simulink model "Lombardy"  (Simulink 7.9)
settings: Solver=ode45  StartTime=0.0  StopTime=10.0  RelTol=1e-3
undefined symbols (not defined in the file or in its folder): f_NODE01, f_NODE02, f_NODE03, f_NODE04, f_NODE05, f_NODE06, f_NODE07, f_NODE08, f_NODE09, f_NODE10, f_NODE11, f_NODE12, f_NODE13, f_NODE14, f_NODE15, f_NODE16, f_NODE17, f_NODE18, f_NODE19, f_NODE20, f_NODE21, f_NODE22, f_NODE23, f_NODE24, f_NODE25, f_NODE26, f_NODE27, f_NODE28, f_NODE29, f_NODE30, f_NODE31, f_NODE32, r_NODE01, r_NODE02, r_NODE03, r_NODE04, r_NODE05, r_NODE06, r_NODE07, r_NODE08, r_NODE09, r_NODE10, r_NODE11, r_NODE12, r_NODE13, r_NODE14, r_NODE15, r_NODE16, r_NODE17, r_NODE18, r_NODE19, r_NODE20, r_NODE21, r_NODE22, r_NODE23, r_NODE24, r_NODE25, r_NODE26, r_NODE27, r_NODE28 ... (+36)
(part 1 of 2)
settings Model: Creator=lanalfa  LastModifiedBy=lanalfa

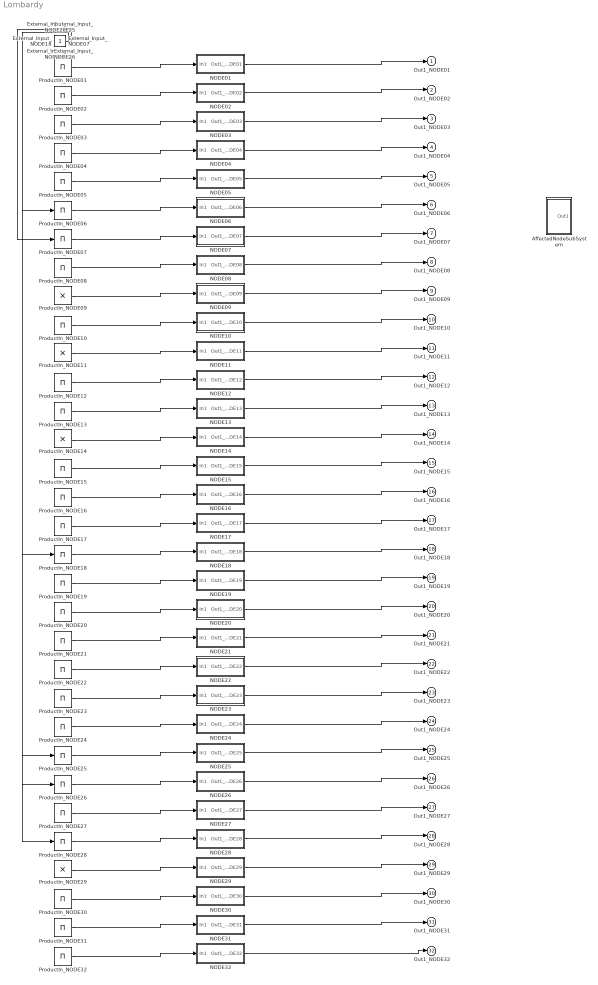
== system Lombardy ==
  AffectedNodeSubSystem : Subsystem
  External_Input_NODE06 : Constant
  External_Input_NODE07 : Constant
  External_Input_NODE{18,25..26,28} (4 alike) : Constant
  NODE01 : Subsystem
  NODE02 : Subsystem
  NODE03 : Subsystem
  NODE04 : Subsystem
  NODE05 : Subsystem
  NODE06 : Subsystem
  NODE07 : Subsystem
  NODE08 : Subsystem
  NODE09 : Subsystem
  NODE10 : Subsystem
  NODE11 : Subsystem
  NODE12 : Subsystem
  NODE13 : Subsystem
  NODE14 : Subsystem
  NODE15 : Subsystem
  NODE16 : Subsystem
  NODE17 : Subsystem
  NODE18 : Subsystem
  NODE19 : Subsystem
  NODE20 : Subsystem
  NODE21 : Subsystem
  NODE22 : Subsystem
  NODE23 : Subsystem
  NODE24 : Subsystem
  NODE25 : Subsystem
  NODE26 : Subsystem
  NODE27 : Subsystem
  NODE28 : Subsystem
  NODE29 : Subsystem
  NODE30 : Subsystem
  NODE31 : Subsystem
  NODE32 : Subsystem
  ProductIn_NODE01 : Product  Inputs=1  SaturateOnIntegerOverflow=on  RndMeth=Zero  InputSameDT=on
  ProductIn_NODE02 : Product  Inputs=1  SaturateOnIntegerOverflow=on  RndMeth=Zero  InputSameDT=on
  ProductIn_NODE03 : Product  Inputs=1  SaturateOnIntegerOverflow=on  RndMeth=Zero  InputSameDT=on
  ProductIn_NODE04 : Product  Inputs=1  SaturateOnIntegerOverflow=on  RndMeth=Zero  InputSameDT=on
  ProductIn_NODE05 : Product  Inputs=1  SaturateOnIntegerOverflow=on  RndMeth=Zero  InputSameDT=on
  ProductIn_NODE06 : Product  Inputs=1  SaturateOnIntegerOverflow=on  RndMeth=Zero  InputSameDT=on
  ProductIn_NODE07 : Product  Inputs=1  SaturateOnIntegerOverflow=on  RndMeth=Zero  InputSameDT=on
  ProductIn_NODE08 : Product  Inputs=1  SaturateOnIntegerOverflow=on  RndMeth=Zero  InputSameDT=on
  ProductIn_NODE09 : Product  SaturateOnIntegerOverflow=on  RndMeth=Zero  InputSameDT=on
  ProductIn_NODE{10,12..13,15..28,30..32} (20 alike) : Product  Inputs=1  SaturateOnIntegerOverflow=on  RndMeth=Zero  InputSameDT=on
  ProductIn_NODE11 : Product  SaturateOnIntegerOverflow=on  RndMeth=Zero  InputSameDT=on
  ProductIn_NODE14 : Product  Inputs=4  SaturateOnIntegerOverflow=on  RndMeth=Zero  InputSameDT=on
  ProductIn_NODE29 : Product  SaturateOnIntegerOverflow=on  RndMeth=Zero  InputSameDT=on
  Out1_NODE01 : Outport
  Out1_NODE02 : Outport  Port=2
  Out1_NODE03 : Outport  Port=3
  Out1_NODE04 : Outport  Port=4
  Out1_NODE05 : Outport  Port=5
  Out1_NODE06 : Outport  Port=6
  Out1_NODE07 : Outport  Port=7
  Out1_NODE08 : Outport  Port=8
  Out1_NODE09 : Outport  Port=9
  Out1_NODE10 : Outport  Port=10
  Out1_NODE11 : Outport  Port=11
  Out1_NODE12 : Outport  Port=12
  Out1_NODE13 : Outport  Port=13
  Out1_NODE14 : Outport  Port=14
  Out1_NODE15 : Outport  Port=15
  Out1_NODE16 : Outport  Port=16
  Out1_NODE17 : Outport  Port=17
  Out1_NODE18 : Outport  Port=18
  Out1_NODE19 : Outport  Port=19
  Out1_NODE20 : Outport  Port=20
  Out1_NODE21 : Outport  Port=21
  Out1_NODE22 : Outport  Port=22
  Out1_NODE23 : Outport  Port=23
  Out1_NODE24 : Outport  Port=24
  Out1_NODE25 : Outport  Port=25
  Out1_NODE26 : Outport  Port=26
  Out1_NODE27 : Outport  Port=27
  Out1_NODE28 : Outport  Port=28
  Out1_NODE29 : Outport  Port=29
  Out1_NODE30 : Outport  Port=30
  Out1_NODE31 : Outport  Port=31
  Out1_NODE32 : Outport  Port=32
  wires:
  ProductIn_NODE01/1 -> NODE01/1(In1)
  NODE01/1(Out1_NODE01) -> Out1_NODE01/1
  ProductIn_NODE02/1 -> NODE02/1(In1)
  NODE02/1(Out1_NODE02) -> Out1_NODE02/1
  ProductIn_NODE03/1 -> NODE03/1(In1)
  NODE03/1(Out1_NODE03) -> Out1_NODE03/1
  ProductIn_NODE04/1 -> NODE04/1(In1)
  NODE04/1(Out1_NODE04) -> Out1_NODE04/1
  ProductIn_NODE05/1 -> NODE05/1(In1)
  NODE05/1(Out1_NODE05) -> Out1_NODE05/1
  ProductIn_NODE06/1 -> NODE06/1(In1)
  NODE06/1(Out1_NODE06) -> Out1_NODE06/1
  ProductIn_NODE07/1 -> NODE07/1(In1)
  NODE07/1(Out1_NODE07) -> Out1_NODE07/1
  ProductIn_NODE08/1 -> NODE08/1(In1)
  NODE08/1(Out1_NODE08) -> Out1_NODE08/1
  ProductIn_NODE09/1 -> NODE09/1(In1)
  NODE09/1(Out1_NODE09) -> Out1_NODE09/1
  ProductIn_NODE10/1 -> NODE10/1(In1)
  NODE10/1(Out1_NODE10) -> Out1_NODE10/1
  ProductIn_NODE11/1 -> NODE11/1(In1)
  NODE11/1(Out1_NODE11) -> Out1_NODE11/1
  ProductIn_NODE12/1 -> NODE12/1(In1)
  NODE12/1(Out1_NODE12) -> Out1_NODE12/1
  ProductIn_NODE13/1 -> NODE13/1(In1)
  NODE13/1(Out1_NODE13) -> Out1_NODE13/1
  ProductIn_NODE14/1 -> NODE14/1(In1)
  NODE14/1(Out1_NODE14) -> Out1_NODE14/1
  ProductIn_NODE15/1 -> NODE15/1(In1)
  NODE15/1(Out1_NODE15) -> Out1_NODE15/1
  ProductIn_NODE16/1 -> NODE16/1(In1)
  NODE16/1(Out1_NODE16) -> Out1_NODE16/1
  ProductIn_NODE17/1 -> NODE17/1(In1)
  NODE17/1(Out1_NODE17) -> Out1_NODE17/1
  ProductIn_NODE18/1 -> NODE18/1(In1)
  NODE18/1(Out1_NODE18) -> Out1_NODE18/1
  ProductIn_NODE19/1 -> NODE19/1(In1)
  NODE19/1(Out1_NODE19) -> Out1_NODE19/1
  ProductIn_NODE20/1 -> NODE20/1(In1)
  NODE20/1(Out1_NODE20) -> Out1_NODE20/1
  ProductIn_NODE21/1 -> NODE21/1(In1)
  NODE21/1(Out1_NODE21) -> Out1_NODE21/1
  ProductIn_NODE22/1 -> NODE22/1(In1)
  NODE22/1(Out1_NODE22) -> Out1_NODE22/1
  ProductIn_NODE23/1 -> NODE23/1(In1)
  NODE23/1(Out1_NODE23) -> Out1_NODE23/1
  ProductIn_NODE24/1 -> NODE24/1(In1)
  NODE24/1(Out1_NODE24) -> Out1_NODE24/1
  ProductIn_NODE25/1 -> NODE25/1(In1)
  NODE25/1(Out1_NODE25) -> Out1_NODE25/1
  ProductIn_NODE26/1 -> NODE26/1(In1)
  NODE26/1(Out1_NODE26) -> Out1_NODE26/1
  ProductIn_NODE27/1 -> NODE27/1(In1)
  NODE27/1(Out1_NODE27) -> Out1_NODE27/1
  ProductIn_NODE28/1 -> NODE28/1(In1)
  NODE28/1(Out1_NODE28) -> Out1_NODE28/1
  ProductIn_NODE29/1 -> NODE29/1(In1)
  NODE29/1(Out1_NODE29) -> Out1_NODE29/1
  ProductIn_NODE30/1 -> NODE30/1(In1)
  NODE30/1(Out1_NODE30) -> Out1_NODE30/1
  ProductIn_NODE31/1 -> NODE31/1(In1)
  NODE31/1(Out1_NODE31) -> Out1_NODE31/1
  ProductIn_NODE32/1 -> NODE32/1(In1)
  NODE32/1(Out1_NODE32) -> Out1_NODE32/1
  External_Input_NODE06/1 -> ProductIn_NODE06/1
  External_Input_NODE07/1 -> ProductIn_NODE07/1
  External_Input_NODE18/1 -> ProductIn_NODE18/1
  External_Input_NODE25/1 -> ProductIn_NODE25/1
  External_Input_NODE26/1 -> ProductIn_NODE26/1
  External_Input_NODE28/1 -> ProductIn_NODE28/1

== system Lombardy/AffectedNodeSubSystem ==
  Pulse Generator_NODE : DiscretePulseGenerator  PulseType=Time based  Period=1  PulseWidth=60  PhaseDelay=0.4
  Out1 : Outport
  wires:
  Pulse Generator_NODE/1 -> Out1/1

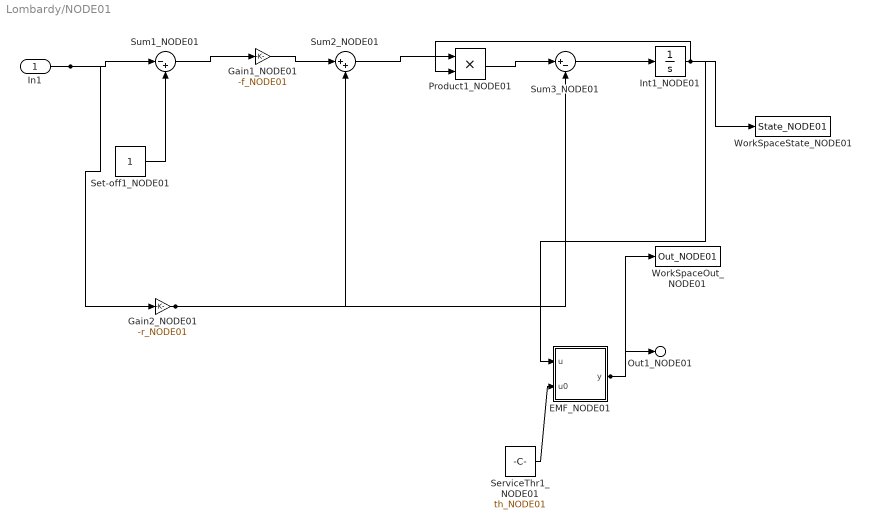
== system Lombardy/NODE01 ==
  In1 : Inport
  EMF_NODE01 : MATLAB Function  TreatAsAtomicUnit=on
  Gain1_NODE01 : Gain  Gain=-f_NODE01  SaturateOnIntegerOverflow=on  OutDataTypeStr=Inherit: Same as input  ParamDataTypeStr=Inherit: Same as input
  Gain2_NODE01 : Gain  Gain=-r_NODE01  SaturateOnIntegerOverflow=on  OutDataTypeStr=Inherit: Same as input  ParamDataTypeStr=Inherit: Same as input
  Int1_NODE01 : Integrator  InitialCondition=1
  Product1_NODE01 : Product  SaturateOnIntegerOverflow=on  RndMeth=Zero  InputSameDT=on
  ServiceThr1_NODE01 : Constant  Value=th_NODE01
  Set-off1_NODE01 : Constant
  Sum1_NODE01 : Sum  Inputs=|-+  SaturateOnIntegerOverflow=on  InputSameDT=on
  Sum2_NODE01 : Sum  Inputs=|++  SaturateOnIntegerOverflow=on  InputSameDT=on
  Sum3_NODE01 : Sum  Inputs=|+-  SaturateOnIntegerOverflow=on  InputSameDT=on
  WorkSpaceOut_NODE01 : ToWorkspace  VariableName=Out_NODE01
  WorkSpaceState_NODE01 : ToWorkspace  VariableName=State_NODE01
  Out1_NODE01 : Outport
  wires:
  In1/1 -> Gain2_NODE01/1, Sum1_NODE01/1
  Set-off1_NODE01/1 -> Sum1_NODE01/2
  Sum1_NODE01/1 -> Gain1_NODE01/1
  Gain1_NODE01/1 -> Sum2_NODE01/1
  Gain2_NODE01/1 -> Sum2_NODE01/2, Sum3_NODE01/2
  Sum2_NODE01/1 -> Product1_NODE01/1
  Product1_NODE01/1 -> Sum3_NODE01/1
  Int1_NODE01/1 -> Product1_NODE01/2, EMF_NODE01/1(u), WorkSpaceState_NODE01/1
  Sum3_NODE01/1 -> Int1_NODE01/1
  ServiceThr1_NODE01/1 -> EMF_NODE01/2(u0)
  EMF_NODE01/1(y) -> Out1_NODE01/1, WorkSpaceOut_NODE01/1

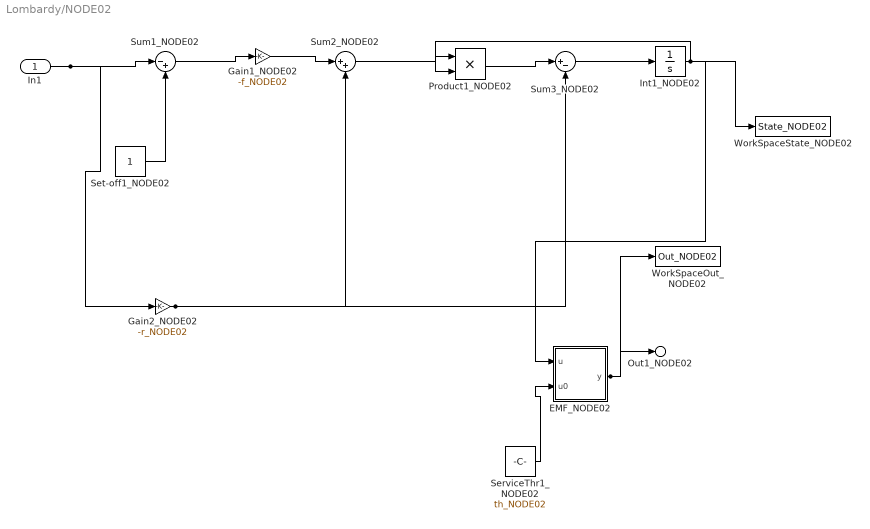
== system Lombardy/NODE02 ==
  In1 : Inport
  EMF_NODE02 : MATLAB Function  TreatAsAtomicUnit=on
  Gain1_NODE02 : Gain  Gain=-f_NODE02  SaturateOnIntegerOverflow=on  OutDataTypeStr=Inherit: Same as input  ParamDataTypeStr=Inherit: Same as input
  Gain2_NODE02 : Gain  Gain=-r_NODE02  SaturateOnIntegerOverflow=on  OutDataTypeStr=Inherit: Same as input  ParamDataTypeStr=Inherit: Same as input
  Int1_NODE02 : Integrator  InitialCondition=1
  Product1_NODE02 : Product  SaturateOnIntegerOverflow=on  RndMeth=Zero  InputSameDT=on
  ServiceThr1_NODE02 : Constant  Value=th_NODE02
  Set-off1_NODE02 : Constant
  Sum1_NODE02 : Sum  Inputs=|-+  SaturateOnIntegerOverflow=on  InputSameDT=on
  Sum2_NODE02 : Sum  Inputs=|++  SaturateOnIntegerOverflow=on  InputSameDT=on
  Sum3_NODE02 : Sum  Inputs=|+-  SaturateOnIntegerOverflow=on  InputSameDT=on
  WorkSpaceOut_NODE02 : ToWorkspace  VariableName=Out_NODE02
  WorkSpaceState_NODE02 : ToWorkspace  VariableName=State_NODE02
  Out1_NODE02 : Outport
  wires:
  In1/1 -> Gain2_NODE02/1, Sum1_NODE02/1
  Set-off1_NODE02/1 -> Sum1_NODE02/2
  Sum1_NODE02/1 -> Gain1_NODE02/1
  Gain1_NODE02/1 -> Sum2_NODE02/1
  Gain2_NODE02/1 -> Sum2_NODE02/2, Sum3_NODE02/2
  Sum2_NODE02/1 -> Product1_NODE02/1
  Product1_NODE02/1 -> Sum3_NODE02/1
  Int1_NODE02/1 -> Product1_NODE02/2, EMF_NODE02/1(u), WorkSpaceState_NODE02/1
  Sum3_NODE02/1 -> Int1_NODE02/1
  ServiceThr1_NODE02/1 -> EMF_NODE02/2(u0)
  EMF_NODE02/1(y) -> Out1_NODE02/1, WorkSpaceOut_NODE02/1

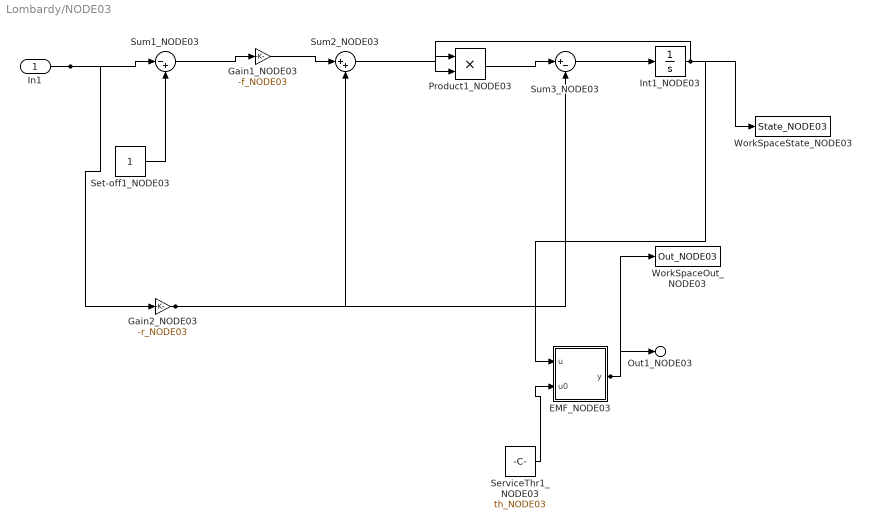
== system Lombardy/NODE03 ==
  In1 : Inport
  EMF_NODE03 : MATLAB Function  TreatAsAtomicUnit=on
  Gain1_NODE03 : Gain  Gain=-f_NODE03  SaturateOnIntegerOverflow=on  OutDataTypeStr=Inherit: Same as input  ParamDataTypeStr=Inherit: Same as input
  Gain2_NODE03 : Gain  Gain=-r_NODE03  SaturateOnIntegerOverflow=on  OutDataTypeStr=Inherit: Same as input  ParamDataTypeStr=Inherit: Same as input
  Int1_NODE03 : Integrator  InitialCondition=1
  Product1_NODE03 : Product  SaturateOnIntegerOverflow=on  RndMeth=Zero  InputSameDT=on
  ServiceThr1_NODE03 : Constant  Value=th_NODE03
  Set-off1_NODE03 : Constant
  Sum1_NODE03 : Sum  Inputs=|-+  SaturateOnIntegerOverflow=on  InputSameDT=on
  Sum2_NODE03 : Sum  Inputs=|++  SaturateOnIntegerOverflow=on  InputSameDT=on
  Sum3_NODE03 : Sum  Inputs=|+-  SaturateOnIntegerOverflow=on  InputSameDT=on
  WorkSpaceOut_NODE03 : ToWorkspace  VariableName=Out_NODE03
  WorkSpaceState_NODE03 : ToWorkspace  VariableName=State_NODE03
  Out1_NODE03 : Outport
  wires:
  In1/1 -> Gain2_NODE03/1, Sum1_NODE03/1
  Set-off1_NODE03/1 -> Sum1_NODE03/2
  Sum1_NODE03/1 -> Gain1_NODE03/1
  Gain1_NODE03/1 -> Sum2_NODE03/1
  Gain2_NODE03/1 -> Sum2_NODE03/2, Sum3_NODE03/2
  Sum2_NODE03/1 -> Product1_NODE03/1
  Product1_NODE03/1 -> Sum3_NODE03/1
  Int1_NODE03/1 -> Product1_NODE03/2, EMF_NODE03/1(u), WorkSpaceState_NODE03/1
  Sum3_NODE03/1 -> Int1_NODE03/1
  ServiceThr1_NODE03/1 -> EMF_NODE03/2(u0)
  EMF_NODE03/1(y) -> Out1_NODE03/1, WorkSpaceOut_NODE03/1

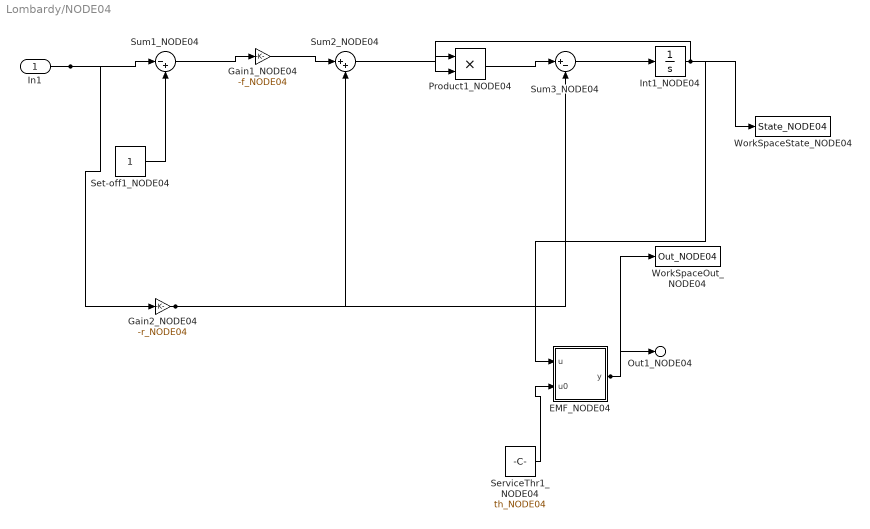
== system Lombardy/NODE04 ==
  In1 : Inport
  EMF_NODE04 : MATLAB Function  TreatAsAtomicUnit=on
  Gain1_NODE04 : Gain  Gain=-f_NODE04  SaturateOnIntegerOverflow=on  OutDataTypeStr=Inherit: Same as input  ParamDataTypeStr=Inherit: Same as input
  Gain2_NODE04 : Gain  Gain=-r_NODE04  SaturateOnIntegerOverflow=on  OutDataTypeStr=Inherit: Same as input  ParamDataTypeStr=Inherit: Same as input
  Int1_NODE04 : Integrator  InitialCondition=1
  Product1_NODE04 : Product  SaturateOnIntegerOverflow=on  RndMeth=Zero  InputSameDT=on
  ServiceThr1_NODE04 : Constant  Value=th_NODE04
  Set-off1_NODE04 : Constant
  Sum1_NODE04 : Sum  Inputs=|-+  SaturateOnIntegerOverflow=on  InputSameDT=on
  Sum2_NODE04 : Sum  Inputs=|++  SaturateOnIntegerOverflow=on  InputSameDT=on
  Sum3_NODE04 : Sum  Inputs=|+-  SaturateOnIntegerOverflow=on  InputSameDT=on
  WorkSpaceOut_NODE04 : ToWorkspace  VariableName=Out_NODE04
  WorkSpaceState_NODE04 : ToWorkspace  VariableName=State_NODE04
  Out1_NODE04 : Outport
  wires:
  In1/1 -> Gain2_NODE04/1, Sum1_NODE04/1
  Set-off1_NODE04/1 -> Sum1_NODE04/2
  Sum1_NODE04/1 -> Gain1_NODE04/1
  Gain1_NODE04/1 -> Sum2_NODE04/1
  Gain2_NODE04/1 -> Sum2_NODE04/2, Sum3_NODE04/2
  Sum2_NODE04/1 -> Product1_NODE04/1
  Product1_NODE04/1 -> Sum3_NODE04/1
  Int1_NODE04/1 -> Product1_NODE04/2, EMF_NODE04/1(u), WorkSpaceState_NODE04/1
  Sum3_NODE04/1 -> Int1_NODE04/1
  ServiceThr1_NODE04/1 -> EMF_NODE04/2(u0)
  EMF_NODE04/1(y) -> Out1_NODE04/1, WorkSpaceOut_NODE04/1

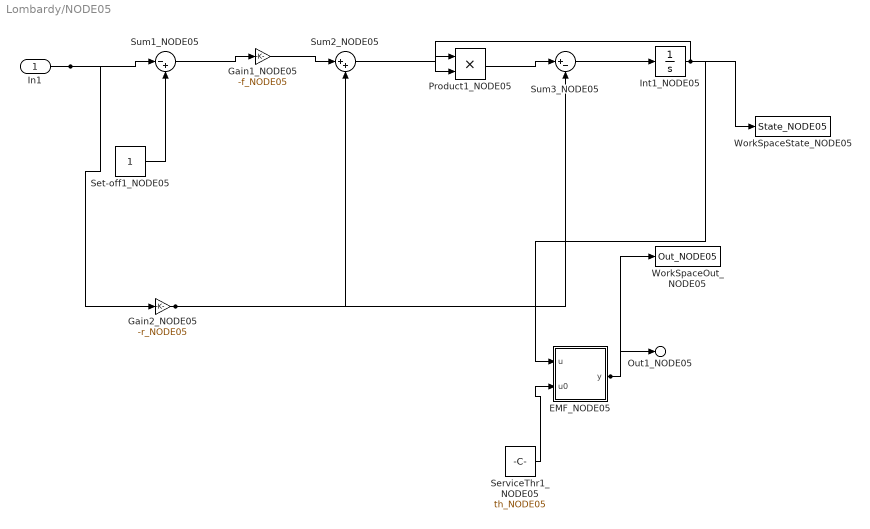
== system Lombardy/NODE05 ==
  In1 : Inport
  EMF_NODE05 : MATLAB Function  TreatAsAtomicUnit=on
  Gain1_NODE05 : Gain  Gain=-f_NODE05  SaturateOnIntegerOverflow=on  OutDataTypeStr=Inherit: Same as input  ParamDataTypeStr=Inherit: Same as input
  Gain2_NODE05 : Gain  Gain=-r_NODE05  SaturateOnIntegerOverflow=on  OutDataTypeStr=Inherit: Same as input  ParamDataTypeStr=Inherit: Same as input
  Int1_NODE05 : Integrator  InitialCondition=1
  Product1_NODE05 : Product  SaturateOnIntegerOverflow=on  RndMeth=Zero  InputSameDT=on
  ServiceThr1_NODE05 : Constant  Value=th_NODE05
  Set-off1_NODE05 : Constant
  Sum1_NODE05 : Sum  Inputs=|-+  SaturateOnIntegerOverflow=on  InputSameDT=on
  Sum2_NODE05 : Sum  Inputs=|++  SaturateOnIntegerOverflow=on  InputSameDT=on
  Sum3_NODE05 : Sum  Inputs=|+-  SaturateOnIntegerOverflow=on  InputSameDT=on
  WorkSpaceOut_NODE05 : ToWorkspace  VariableName=Out_NODE05
  WorkSpaceState_NODE05 : ToWorkspace  VariableName=State_NODE05
  Out1_NODE05 : Outport
  wires:
  In1/1 -> Gain2_NODE05/1, Sum1_NODE05/1
  Set-off1_NODE05/1 -> Sum1_NODE05/2
  Sum1_NODE05/1 -> Gain1_NODE05/1
  Gain1_NODE05/1 -> Sum2_NODE05/1
  Gain2_NODE05/1 -> Sum2_NODE05/2, Sum3_NODE05/2
  Sum2_NODE05/1 -> Product1_NODE05/1
  Product1_NODE05/1 -> Sum3_NODE05/1
  Int1_NODE05/1 -> Product1_NODE05/2, EMF_NODE05/1(u), WorkSpaceState_NODE05/1
  Sum3_NODE05/1 -> Int1_NODE05/1
  ServiceThr1_NODE05/1 -> EMF_NODE05/2(u0)
  EMF_NODE05/1(y) -> Out1_NODE05/1, WorkSpaceOut_NODE05/1

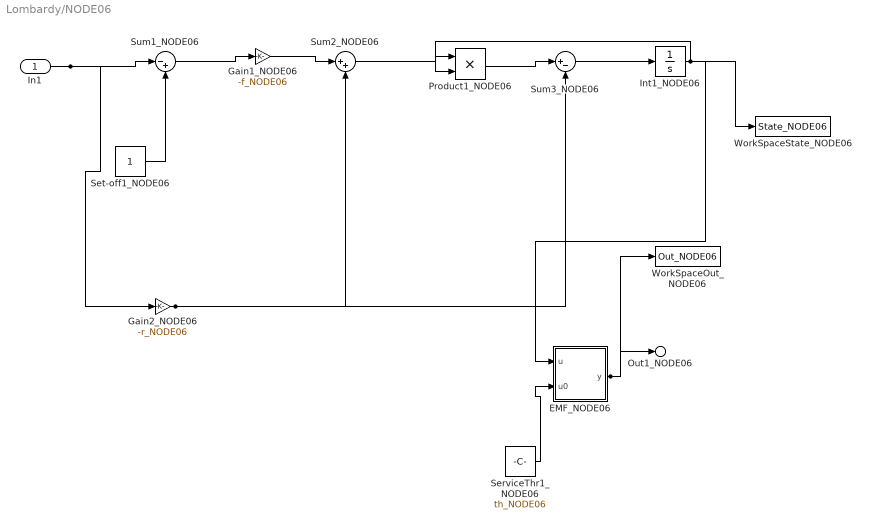
== system Lombardy/NODE06 ==
  In1 : Inport
  EMF_NODE06 : MATLAB Function  TreatAsAtomicUnit=on
  Gain1_NODE06 : Gain  Gain=-f_NODE06  SaturateOnIntegerOverflow=on  OutDataTypeStr=Inherit: Same as input  ParamDataTypeStr=Inherit: Same as input
  Gain2_NODE06 : Gain  Gain=-r_NODE06  SaturateOnIntegerOverflow=on  OutDataTypeStr=Inherit: Same as input  ParamDataTypeStr=Inherit: Same as input
  Int1_NODE06 : Integrator  InitialCondition=1
  Product1_NODE06 : Product  SaturateOnIntegerOverflow=on  RndMeth=Zero  InputSameDT=on
  ServiceThr1_NODE06 : Constant  Value=th_NODE06
  Set-off1_NODE06 : Constant
  Sum1_NODE06 : Sum  Inputs=|-+  SaturateOnIntegerOverflow=on  InputSameDT=on
  Sum2_NODE06 : Sum  Inputs=|++  SaturateOnIntegerOverflow=on  InputSameDT=on
  Sum3_NODE06 : Sum  Inputs=|+-  SaturateOnIntegerOverflow=on  InputSameDT=on
  WorkSpaceOut_NODE06 : ToWorkspace  VariableName=Out_NODE06
  WorkSpaceState_NODE06 : ToWorkspace  VariableName=State_NODE06
  Out1_NODE06 : Outport
  wires:
  In1/1 -> Gain2_NODE06/1, Sum1_NODE06/1
  Set-off1_NODE06/1 -> Sum1_NODE06/2
  Sum1_NODE06/1 -> Gain1_NODE06/1
  Gain1_NODE06/1 -> Sum2_NODE06/1
  Gain2_NODE06/1 -> Sum2_NODE06/2, Sum3_NODE06/2
  Sum2_NODE06/1 -> Product1_NODE06/1
  Product1_NODE06/1 -> Sum3_NODE06/1
  Int1_NODE06/1 -> Product1_NODE06/2, EMF_NODE06/1(u), WorkSpaceState_NODE06/1
  Sum3_NODE06/1 -> Int1_NODE06/1
  ServiceThr1_NODE06/1 -> EMF_NODE06/2(u0)
  EMF_NODE06/1(y) -> Out1_NODE06/1, WorkSpaceOut_NODE06/1

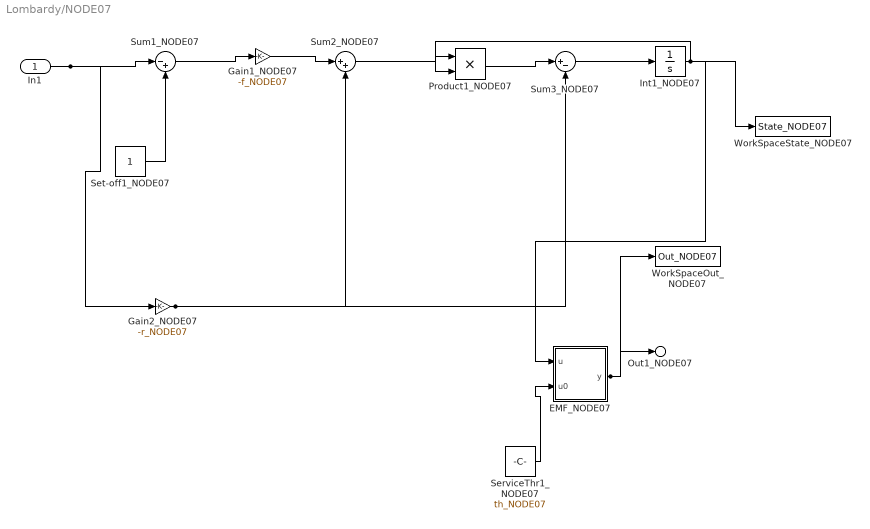
== system Lombardy/NODE07 ==
  In1 : Inport
  EMF_NODE07 : MATLAB Function  TreatAsAtomicUnit=on
  Gain1_NODE07 : Gain  Gain=-f_NODE07  SaturateOnIntegerOverflow=on  OutDataTypeStr=Inherit: Same as input  ParamDataTypeStr=Inherit: Same as input
  Gain2_NODE07 : Gain  Gain=-r_NODE07  SaturateOnIntegerOverflow=on  OutDataTypeStr=Inherit: Same as input  ParamDataTypeStr=Inherit: Same as input
  Int1_NODE07 : Integrator  InitialCondition=1
  Product1_NODE07 : Product  SaturateOnIntegerOverflow=on  RndMeth=Zero  InputSameDT=on
  ServiceThr1_NODE07 : Constant  Value=th_NODE07
  Set-off1_NODE07 : Constant
  Sum1_NODE07 : Sum  Inputs=|-+  SaturateOnIntegerOverflow=on  InputSameDT=on
  Sum2_NODE07 : Sum  Inputs=|++  SaturateOnIntegerOverflow=on  InputSameDT=on
  Sum3_NODE07 : Sum  Inputs=|+-  SaturateOnIntegerOverflow=on  InputSameDT=on
  WorkSpaceOut_NODE07 : ToWorkspace  VariableName=Out_NODE07
  WorkSpaceState_NODE07 : ToWorkspace  VariableName=State_NODE07
  Out1_NODE07 : Outport
  wires:
  In1/1 -> Gain2_NODE07/1, Sum1_NODE07/1
  Set-off1_NODE07/1 -> Sum1_NODE07/2
  Sum1_NODE07/1 -> Gain1_NODE07/1
  Gain1_NODE07/1 -> Sum2_NODE07/1
  Gain2_NODE07/1 -> Sum2_NODE07/2, Sum3_NODE07/2
  Sum2_NODE07/1 -> Product1_NODE07/1
  Product1_NODE07/1 -> Sum3_NODE07/1
  Int1_NODE07/1 -> Product1_NODE07/2, EMF_NODE07/1(u), WorkSpaceState_NODE07/1
  Sum3_NODE07/1 -> Int1_NODE07/1
  ServiceThr1_NODE07/1 -> EMF_NODE07/2(u0)
  EMF_NODE07/1(y) -> Out1_NODE07/1, WorkSpaceOut_NODE07/1

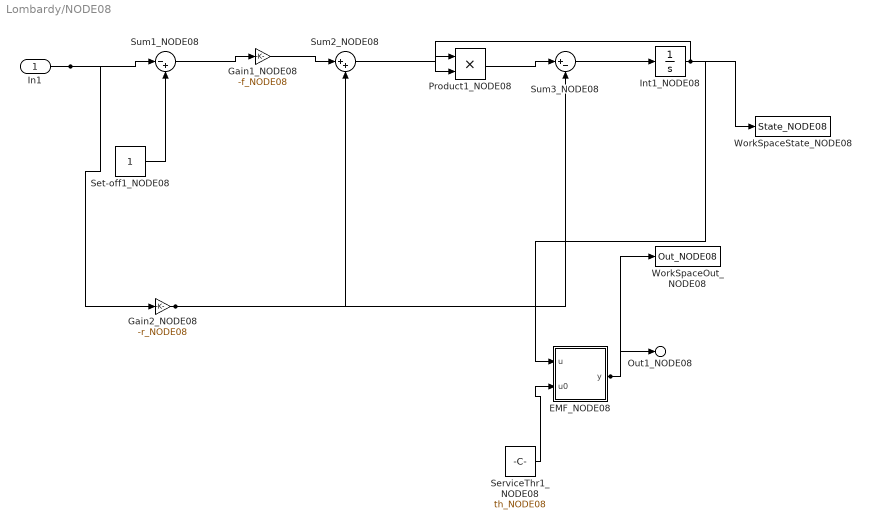
== system Lombardy/NODE08 ==
  In1 : Inport
  EMF_NODE08 : MATLAB Function  TreatAsAtomicUnit=on
  Gain1_NODE08 : Gain  Gain=-f_NODE08  SaturateOnIntegerOverflow=on  OutDataTypeStr=Inherit: Same as input  ParamDataTypeStr=Inherit: Same as input
  Gain2_NODE08 : Gain  Gain=-r_NODE08  SaturateOnIntegerOverflow=on  OutDataTypeStr=Inherit: Same as input  ParamDataTypeStr=Inherit: Same as input
  Int1_NODE08 : Integrator  InitialCondition=1
  Product1_NODE08 : Product  SaturateOnIntegerOverflow=on  RndMeth=Zero  InputSameDT=on
  ServiceThr1_NODE08 : Constant  Value=th_NODE08
  Set-off1_NODE08 : Constant
  Sum1_NODE08 : Sum  Inputs=|-+  SaturateOnIntegerOverflow=on  InputSameDT=on
  Sum2_NODE08 : Sum  Inputs=|++  SaturateOnIntegerOverflow=on  InputSameDT=on
  Sum3_NODE08 : Sum  Inputs=|+-  SaturateOnIntegerOverflow=on  InputSameDT=on
  WorkSpaceOut_NODE08 : ToWorkspace  VariableName=Out_NODE08
  WorkSpaceState_NODE08 : ToWorkspace  VariableName=State_NODE08
  Out1_NODE08 : Outport
  wires:
  In1/1 -> Gain2_NODE08/1, Sum1_NODE08/1
  Set-off1_NODE08/1 -> Sum1_NODE08/2
  Sum1_NODE08/1 -> Gain1_NODE08/1
  Gain1_NODE08/1 -> Sum2_NODE08/1
  Gain2_NODE08/1 -> Sum2_NODE08/2, Sum3_NODE08/2
  Sum2_NODE08/1 -> Product1_NODE08/1
  Product1_NODE08/1 -> Sum3_NODE08/1
  Int1_NODE08/1 -> Product1_NODE08/2, EMF_NODE08/1(u), WorkSpaceState_NODE08/1
  Sum3_NODE08/1 -> Int1_NODE08/1
  ServiceThr1_NODE08/1 -> EMF_NODE08/2(u0)
  EMF_NODE08/1(y) -> Out1_NODE08/1, WorkSpaceOut_NODE08/1

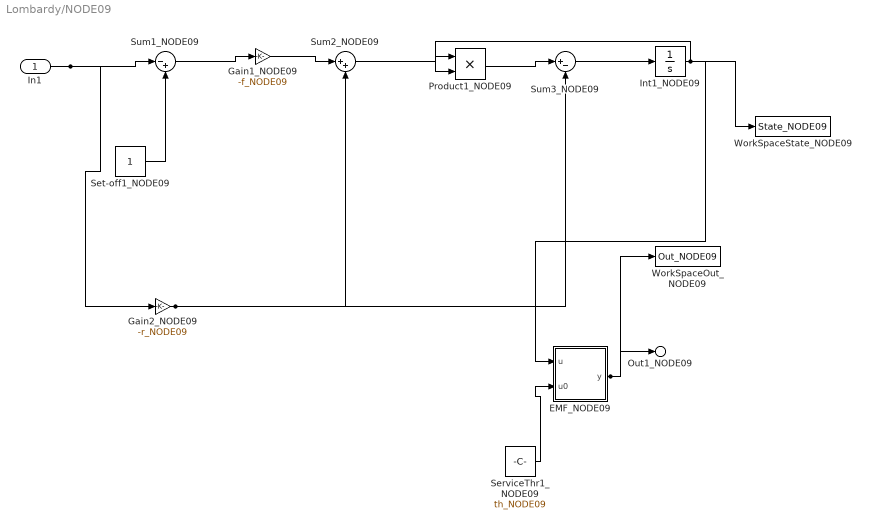
== system Lombardy/NODE09 ==
  In1 : Inport
  EMF_NODE09 : MATLAB Function  TreatAsAtomicUnit=on
  Gain1_NODE09 : Gain  Gain=-f_NODE09  SaturateOnIntegerOverflow=on  OutDataTypeStr=Inherit: Same as input  ParamDataTypeStr=Inherit: Same as input
  Gain2_NODE09 : Gain  Gain=-r_NODE09  SaturateOnIntegerOverflow=on  OutDataTypeStr=Inherit: Same as input  ParamDataTypeStr=Inherit: Same as input
  Int1_NODE09 : Integrator  InitialCondition=1
  Product1_NODE09 : Product  SaturateOnIntegerOverflow=on  RndMeth=Zero  InputSameDT=on
  ServiceThr1_NODE09 : Constant  Value=th_NODE09
  Set-off1_NODE09 : Constant
  Sum1_NODE09 : Sum  Inputs=|-+  SaturateOnIntegerOverflow=on  InputSameDT=on
  Sum2_NODE09 : Sum  Inputs=|++  SaturateOnIntegerOverflow=on  InputSameDT=on
  Sum3_NODE09 : Sum  Inputs=|+-  SaturateOnIntegerOverflow=on  InputSameDT=on
  WorkSpaceOut_NODE09 : ToWorkspace  VariableName=Out_NODE09
  WorkSpaceState_NODE09 : ToWorkspace  VariableName=State_NODE09
  Out1_NODE09 : Outport
  wires:
  In1/1 -> Gain2_NODE09/1, Sum1_NODE09/1
  Set-off1_NODE09/1 -> Sum1_NODE09/2
  Sum1_NODE09/1 -> Gain1_NODE09/1
  Gain1_NODE09/1 -> Sum2_NODE09/1
  Gain2_NODE09/1 -> Sum2_NODE09/2, Sum3_NODE09/2
  Sum2_NODE09/1 -> Product1_NODE09/1
  Product1_NODE09/1 -> Sum3_NODE09/1
  Int1_NODE09/1 -> Product1_NODE09/2, EMF_NODE09/1(u), WorkSpaceState_NODE09/1
  Sum3_NODE09/1 -> Int1_NODE09/1
  ServiceThr1_NODE09/1 -> EMF_NODE09/2(u0)
  EMF_NODE09/1(y) -> Out1_NODE09/1, WorkSpaceOut_NODE09/1

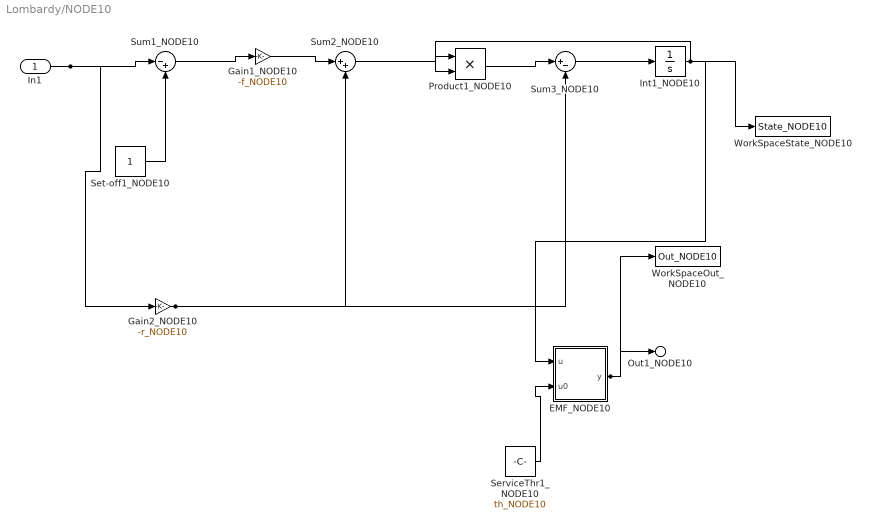
== system Lombardy/NODE10 ==
  In1 : Inport
  EMF_NODE10 : MATLAB Function  TreatAsAtomicUnit=on
  Gain1_NODE10 : Gain  Gain=-f_NODE10  SaturateOnIntegerOverflow=on  OutDataTypeStr=Inherit: Same as input  ParamDataTypeStr=Inherit: Same as input
  Gain2_NODE10 : Gain  Gain=-r_NODE10  SaturateOnIntegerOverflow=on  OutDataTypeStr=Inherit: Same as input  ParamDataTypeStr=Inherit: Same as input
  Int1_NODE10 : Integrator  InitialCondition=1
  Product1_NODE10 : Product  SaturateOnIntegerOverflow=on  RndMeth=Zero  InputSameDT=on
  ServiceThr1_NODE10 : Constant  Value=th_NODE10
  Set-off1_NODE10 : Constant
  Sum1_NODE10 : Sum  Inputs=|-+  SaturateOnIntegerOverflow=on  InputSameDT=on
  Sum2_NODE10 : Sum  Inputs=|++  SaturateOnIntegerOverflow=on  InputSameDT=on
  Sum3_NODE10 : Sum  Inputs=|+-  SaturateOnIntegerOverflow=on  InputSameDT=on
  WorkSpaceOut_NODE10 : ToWorkspace  VariableName=Out_NODE10
  WorkSpaceState_NODE10 : ToWorkspace  VariableName=State_NODE10
  Out1_NODE10 : Outport
  wires:
  In1/1 -> Gain2_NODE10/1, Sum1_NODE10/1
  Set-off1_NODE10/1 -> Sum1_NODE10/2
  Sum1_NODE10/1 -> Gain1_NODE10/1
  Gain1_NODE10/1 -> Sum2_NODE10/1
  Gain2_NODE10/1 -> Sum2_NODE10/2, Sum3_NODE10/2
  Sum2_NODE10/1 -> Product1_NODE10/1
  Product1_NODE10/1 -> Sum3_NODE10/1
  Int1_NODE10/1 -> Product1_NODE10/2, EMF_NODE10/1(u), WorkSpaceState_NODE10/1
  Sum3_NODE10/1 -> Int1_NODE10/1
  ServiceThr1_NODE10/1 -> EMF_NODE10/2(u0)
  EMF_NODE10/1(y) -> Out1_NODE10/1, WorkSpaceOut_NODE10/1

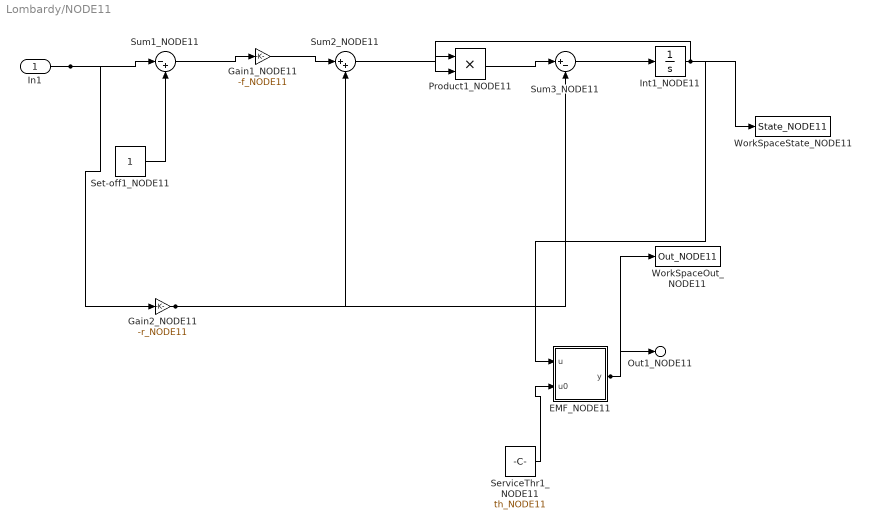
== system Lombardy/NODE11 ==
  In1 : Inport
  EMF_NODE11 : MATLAB Function  TreatAsAtomicUnit=on
  Gain1_NODE11 : Gain  Gain=-f_NODE11  SaturateOnIntegerOverflow=on  OutDataTypeStr=Inherit: Same as input  ParamDataTypeStr=Inherit: Same as input
  Gain2_NODE11 : Gain  Gain=-r_NODE11  SaturateOnIntegerOverflow=on  OutDataTypeStr=Inherit: Same as input  ParamDataTypeStr=Inherit: Same as input
  Int1_NODE11 : Integrator  InitialCondition=1
  Product1_NODE11 : Product  SaturateOnIntegerOverflow=on  RndMeth=Zero  InputSameDT=on
  ServiceThr1_NODE11 : Constant  Value=th_NODE11
  Set-off1_NODE11 : Constant
  Sum1_NODE11 : Sum  Inputs=|-+  SaturateOnIntegerOverflow=on  InputSameDT=on
  Sum2_NODE11 : Sum  Inputs=|++  SaturateOnIntegerOverflow=on  InputSameDT=on
  Sum3_NODE11 : Sum  Inputs=|+-  SaturateOnIntegerOverflow=on  InputSameDT=on
  WorkSpaceOut_NODE11 : ToWorkspace  VariableName=Out_NODE11
  WorkSpaceState_NODE11 : ToWorkspace  VariableName=State_NODE11
  Out1_NODE11 : Outport
  wires:
  In1/1 -> Gain2_NODE11/1, Sum1_NODE11/1
  Set-off1_NODE11/1 -> Sum1_NODE11/2
  Sum1_NODE11/1 -> Gain1_NODE11/1
  Gain1_NODE11/1 -> Sum2_NODE11/1
  Gain2_NODE11/1 -> Sum2_NODE11/2, Sum3_NODE11/2
  Sum2_NODE11/1 -> Product1_NODE11/1
  Product1_NODE11/1 -> Sum3_NODE11/1
  Int1_NODE11/1 -> Product1_NODE11/2, EMF_NODE11/1(u), WorkSpaceState_NODE11/1
  Sum3_NODE11/1 -> Int1_NODE11/1
  ServiceThr1_NODE11/1 -> EMF_NODE11/2(u0)
  EMF_NODE11/1(y) -> Out1_NODE11/1, WorkSpaceOut_NODE11/1

== system Lombardy/NODE12 ==
  In1 : Inport
  EMF_NODE12 : MATLAB Function  TreatAsAtomicUnit=on
  Gain1_NODE12 : Gain  Gain=-f_NODE12  SaturateOnIntegerOverflow=on  OutDataTypeStr=Inherit: Same as input  ParamDataTypeStr=Inherit: Same as input
  Gain2_NODE12 : Gain  Gain=-r_NODE12  SaturateOnIntegerOverflow=on  OutDataTypeStr=Inherit: Same as input  ParamDataTypeStr=Inherit: Same as input
  Int1_NODE12 : Integrator  InitialCondition=1
  Product1_NODE12 : Product  SaturateOnIntegerOverflow=on  RndMeth=Zero  InputSameDT=on
  ServiceThr1_NODE12 : Constant  Value=th_NODE12
  Set-off1_NODE12 : Constant
  Sum1_NODE12 : Sum  Inputs=|-+  SaturateOnIntegerOverflow=on  InputSameDT=on
  Sum2_NODE12 : Sum  Inputs=|++  SaturateOnIntegerOverflow=on  InputSameDT=on
  Sum3_NODE12 : Sum  Inputs=|+-  SaturateOnIntegerOverflow=on  InputSameDT=on
  WorkSpaceOut_NODE12 : ToWorkspace  VariableName=Out_NODE12
  WorkSpaceState_NODE12 : ToWorkspace  VariableName=State_NODE12
  Out1_NODE12 : Outport
  wires:
  In1/1 -> Gain2_NODE12/1, Sum1_NODE12/1
  Set-off1_NODE12/1 -> Sum1_NODE12/2
  Sum1_NODE12/1 -> Gain1_NODE12/1
  Gain1_NODE12/1 -> Sum2_NODE12/1
  Gain2_NODE12/1 -> Sum2_NODE12/2, Sum3_NODE12/2
  Sum2_NODE12/1 -> Product1_NODE12/1
  Product1_NODE12/1 -> Sum3_NODE12/1
  Int1_NODE12/1 -> Product1_NODE12/2, EMF_NODE12/1(u), WorkSpaceState_NODE12/1
  Sum3_NODE12/1 -> Int1_NODE12/1
  ServiceThr1_NODE12/1 -> EMF_NODE12/2(u0)
  EMF_NODE12/1(y) -> Out1_NODE12/1, WorkSpaceOut_NODE12/1

== system Lombardy/NODE13 ==
  In1 : Inport
  EMF_NODE13 : MATLAB Function  TreatAsAtomicUnit=on
  Gain1_NODE13 : Gain  Gain=-f_NODE13  SaturateOnIntegerOverflow=on  OutDataTypeStr=Inherit: Same as input  ParamDataTypeStr=Inherit: Same as input
  Gain2_NODE13 : Gain  Gain=-r_NODE13  SaturateOnIntegerOverflow=on  OutDataTypeStr=Inherit: Same as input  ParamDataTypeStr=Inherit: Same as input
  Int1_NODE13 : Integrator  InitialCondition=1
  Product1_NODE13 : Product  SaturateOnIntegerOverflow=on  RndMeth=Zero  InputSameDT=on
  ServiceThr1_NODE13 : Constant  Value=th_NODE13
  Set-off1_NODE13 : Constant
  Sum1_NODE13 : Sum  Inputs=|-+  SaturateOnIntegerOverflow=on  InputSameDT=on
  Sum2_NODE13 : Sum  Inputs=|++  SaturateOnIntegerOverflow=on  InputSameDT=on
  Sum3_NODE13 : Sum  Inputs=|+-  SaturateOnIntegerOverflow=on  InputSameDT=on
  WorkSpaceOut_NODE13 : ToWorkspace  VariableName=Out_NODE13
  WorkSpaceState_NODE13 : ToWorkspace  VariableName=State_NODE13
  Out1_NODE13 : Outport
  wires:
  In1/1 -> Gain2_NODE13/1, Sum1_NODE13/1
  Set-off1_NODE13/1 -> Sum1_NODE13/2
  Sum1_NODE13/1 -> Gain1_NODE13/1
  Gain1_NODE13/1 -> Sum2_NODE13/1
  Gain2_NODE13/1 -> Sum2_NODE13/2, Sum3_NODE13/2
  Sum2_NODE13/1 -> Product1_NODE13/1
  Product1_NODE13/1 -> Sum3_NODE13/1
  Int1_NODE13/1 -> Product1_NODE13/2, EMF_NODE13/1(u), WorkSpaceState_NODE13/1
  Sum3_NODE13/1 -> Int1_NODE13/1
  ServiceThr1_NODE13/1 -> EMF_NODE13/2(u0)
  EMF_NODE13/1(y) -> Out1_NODE13/1, WorkSpaceOut_NODE13/1

== system Lombardy/NODE14 ==
  In1 : Inport
  EMF_NODE14 : MATLAB Function  TreatAsAtomicUnit=on
  Gain1_NODE14 : Gain  Gain=-f_NODE14  SaturateOnIntegerOverflow=on  OutDataTypeStr=Inherit: Same as input  ParamDataTypeStr=Inherit: Same as input
  Gain2_NODE14 : Gain  Gain=-r_NODE14  SaturateOnIntegerOverflow=on  OutDataTypeStr=Inherit: Same as input  ParamDataTypeStr=Inherit: Same as input
  Int1_NODE14 : Integrator  InitialCondition=1
  Product1_NODE14 : Product  SaturateOnIntegerOverflow=on  RndMeth=Zero  InputSameDT=on
  ServiceThr1_NODE14 : Constant  Value=th_NODE14
  Set-off1_NODE14 : Constant
  Sum1_NODE14 : Sum  Inputs=|-+  SaturateOnIntegerOverflow=on  InputSameDT=on
  Sum2_NODE14 : Sum  Inputs=|++  SaturateOnIntegerOverflow=on  InputSameDT=on
  Sum3_NODE14 : Sum  Inputs=|+-  SaturateOnIntegerOverflow=on  InputSameDT=on
  WorkSpaceOut_NODE14 : ToWorkspace  VariableName=Out_NODE14
  WorkSpaceState_NODE14 : ToWorkspace  VariableName=State_NODE14
  Out1_NODE14 : Outport
  wires:
  In1/1 -> Gain2_NODE14/1, Sum1_NODE14/1
  Set-off1_NODE14/1 -> Sum1_NODE14/2
  Sum1_NODE14/1 -> Gain1_NODE14/1
  Gain1_NODE14/1 -> Sum2_NODE14/1
  Gain2_NODE14/1 -> Sum2_NODE14/2, Sum3_NODE14/2
  Sum2_NODE14/1 -> Product1_NODE14/1
  Product1_NODE14/1 -> Sum3_NODE14/1
  Int1_NODE14/1 -> Product1_NODE14/2, EMF_NODE14/1(u), WorkSpaceState_NODE14/1
  Sum3_NODE14/1 -> Int1_NODE14/1
  ServiceThr1_NODE14/1 -> EMF_NODE14/2(u0)
  EMF_NODE14/1(y) -> Out1_NODE14/1, WorkSpaceOut_NODE14/1

== system Lombardy/NODE15 ==
  In1 : Inport
  EMF_NODE15 : MATLAB Function  TreatAsAtomicUnit=on
  Gain1_NODE15 : Gain  Gain=-f_NODE15  SaturateOnIntegerOverflow=on  OutDataTypeStr=Inherit: Same as input  ParamDataTypeStr=Inherit: Same as input
  Gain2_NODE15 : Gain  Gain=-r_NODE15  SaturateOnIntegerOverflow=on  OutDataTypeStr=Inherit: Same as input  ParamDataTypeStr=Inherit: Same as input
  Int1_NODE15 : Integrator  InitialCondition=1
  Product1_NODE15 : Product  SaturateOnIntegerOverflow=on  RndMeth=Zero  InputSameDT=on
  ServiceThr1_NODE15 : Constant  Value=th_NODE15
  Set-off1_NODE15 : Constant
  Sum1_NODE15 : Sum  Inputs=|-+  SaturateOnIntegerOverflow=on  InputSameDT=on
  Sum2_NODE15 : Sum  Inputs=|++  SaturateOnIntegerOverflow=on  InputSameDT=on
  Sum3_NODE15 : Sum  Inputs=|+-  SaturateOnIntegerOverflow=on  InputSameDT=on
  WorkSpaceOut_NODE15 : ToWorkspace  VariableName=Out_NODE15
  WorkSpaceState_NODE15 : ToWorkspace  VariableName=State_NODE15
  Out1_NODE15 : Outport
  wires:
  In1/1 -> Gain2_NODE15/1, Sum1_NODE15/1
  Set-off1_NODE15/1 -> Sum1_NODE15/2
  Sum1_NODE15/1 -> Gain1_NODE15/1
  Gain1_NODE15/1 -> Sum2_NODE15/1
  Gain2_NODE15/1 -> Sum2_NODE15/2, Sum3_NODE15/2
  Sum2_NODE15/1 -> Product1_NODE15/1
  Product1_NODE15/1 -> Sum3_NODE15/1
  Int1_NODE15/1 -> Product1_NODE15/2, EMF_NODE15/1(u), WorkSpaceState_NODE15/1
  Sum3_NODE15/1 -> Int1_NODE15/1
  ServiceThr1_NODE15/1 -> EMF_NODE15/2(u0)
  EMF_NODE15/1(y) -> Out1_NODE15/1, WorkSpaceOut_NODE15/1

== system Lombardy/NODE16 ==
  In1 : Inport
  EMF_NODE16 : MATLAB Function  TreatAsAtomicUnit=on
  Gain1_NODE16 : Gain  Gain=-f_NODE16  SaturateOnIntegerOverflow=on  OutDataTypeStr=Inherit: Same as input  ParamDataTypeStr=Inherit: Same as input
  Gain2_NODE16 : Gain  Gain=-r_NODE16  SaturateOnIntegerOverflow=on  OutDataTypeStr=Inherit: Same as input  ParamDataTypeStr=Inherit: Same as input
  Int1_NODE16 : Integrator  InitialCondition=1
  Product1_NODE16 : Product  SaturateOnIntegerOverflow=on  RndMeth=Zero  InputSameDT=on
  ServiceThr1_NODE16 : Constant  Value=th_NODE16
  Set-off1_NODE16 : Constant
  Sum1_NODE16 : Sum  Inputs=|-+  SaturateOnIntegerOverflow=on  InputSameDT=on
  Sum2_NODE16 : Sum  Inputs=|++  SaturateOnIntegerOverflow=on  InputSameDT=on
  Sum3_NODE16 : Sum  Inputs=|+-  SaturateOnIntegerOverflow=on  InputSameDT=on
  WorkSpaceOut_NODE16 : ToWorkspace  VariableName=Out_NODE16
  WorkSpaceState_NODE16 : ToWorkspace  VariableName=State_NODE16
  Out1_NODE16 : Outport
  wires:
  In1/1 -> Gain2_NODE16/1, Sum1_NODE16/1
  Set-off1_NODE16/1 -> Sum1_NODE16/2
  Sum1_NODE16/1 -> Gain1_NODE16/1
  Gain1_NODE16/1 -> Sum2_NODE16/1
  Gain2_NODE16/1 -> Sum2_NODE16/2, Sum3_NODE16/2
  Sum2_NODE16/1 -> Product1_NODE16/1
  Product1_NODE16/1 -> Sum3_NODE16/1
  Int1_NODE16/1 -> Product1_NODE16/2, EMF_NODE16/1(u), WorkSpaceState_NODE16/1
  Sum3_NODE16/1 -> Int1_NODE16/1
  ServiceThr1_NODE16/1 -> EMF_NODE16/2(u0)
  EMF_NODE16/1(y) -> Out1_NODE16/1, WorkSpaceOut_NODE16/1

== system Lombardy/NODE17 ==
  In1 : Inport
  EMF_NODE17 : MATLAB Function  TreatAsAtomicUnit=on
  Gain1_NODE17 : Gain  Gain=-f_NODE17  SaturateOnIntegerOverflow=on  OutDataTypeStr=Inherit: Same as input  ParamDataTypeStr=Inherit: Same as input
  Gain2_NODE17 : Gain  Gain=-r_NODE17  SaturateOnIntegerOverflow=on  OutDataTypeStr=Inherit: Same as input  ParamDataTypeStr=Inherit: Same as input
  Int1_NODE17 : Integrator  InitialCondition=1
  Product1_NODE17 : Product  SaturateOnIntegerOverflow=on  RndMeth=Zero  InputSameDT=on
  ServiceThr1_NODE17 : Constant  Value=th_NODE17
  Set-off1_NODE17 : Constant
  Sum1_NODE17 : Sum  Inputs=|-+  SaturateOnIntegerOverflow=on  InputSameDT=on
  Sum2_NODE17 : Sum  Inputs=|++  SaturateOnIntegerOverflow=on  InputSameDT=on
  Sum3_NODE17 : Sum  Inputs=|+-  SaturateOnIntegerOverflow=on  InputSameDT=on
  WorkSpaceOut_NODE17 : ToWorkspace  VariableName=Out_NODE17
  WorkSpaceState_NODE17 : ToWorkspace  VariableName=State_NODE17
  Out1_NODE17 : Outport
  wires:
  In1/1 -> Gain2_NODE17/1, Sum1_NODE17/1
  Set-off1_NODE17/1 -> Sum1_NODE17/2
  Sum1_NODE17/1 -> Gain1_NODE17/1
  Gain1_NODE17/1 -> Sum2_NODE17/1
  Gain2_NODE17/1 -> Sum2_NODE17/2, Sum3_NODE17/2
  Sum2_NODE17/1 -> Product1_NODE17/1
  Product1_NODE17/1 -> Sum3_NODE17/1
  Int1_NODE17/1 -> Product1_NODE17/2, EMF_NODE17/1(u), WorkSpaceState_NODE17/1
  Sum3_NODE17/1 -> Int1_NODE17/1
  ServiceThr1_NODE17/1 -> EMF_NODE17/2(u0)
  EMF_NODE17/1(y) -> Out1_NODE17/1, WorkSpaceOut_NODE17/1

== system Lombardy/NODE18 ==
  In1 : Inport
  EMF_NODE18 : MATLAB Function  TreatAsAtomicUnit=on
  Gain1_NODE18 : Gain  Gain=-f_NODE18  SaturateOnIntegerOverflow=on  OutDataTypeStr=Inherit: Same as input  ParamDataTypeStr=Inherit: Same as input
  Gain2_NODE18 : Gain  Gain=-r_NODE18  SaturateOnIntegerOverflow=on  OutDataTypeStr=Inherit: Same as input  ParamDataTypeStr=Inherit: Same as input
  Int1_NODE18 : Integrator  InitialCondition=1
  Product1_NODE18 : Product  SaturateOnIntegerOverflow=on  RndMeth=Zero  InputSameDT=on
  ServiceThr1_NODE18 : Constant  Value=th_NODE18
  Set-off1_NODE18 : Constant
  Sum1_NODE18 : Sum  Inputs=|-+  SaturateOnIntegerOverflow=on  InputSameDT=on
  Sum2_NODE18 : Sum  Inputs=|++  SaturateOnIntegerOverflow=on  InputSameDT=on
  Sum3_NODE18 : Sum  Inputs=|+-  SaturateOnIntegerOverflow=on  InputSameDT=on
  WorkSpaceOut_NODE18 : ToWorkspace  VariableName=Out_NODE18
  WorkSpaceState_NODE18 : ToWorkspace  VariableName=State_NODE18
  Out1_NODE18 : Outport
  wires:
  In1/1 -> Gain2_NODE18/1, Sum1_NODE18/1
  Set-off1_NODE18/1 -> Sum1_NODE18/2
  Sum1_NODE18/1 -> Gain1_NODE18/1
  Gain1_NODE18/1 -> Sum2_NODE18/1
  Gain2_NODE18/1 -> Sum2_NODE18/2, Sum3_NODE18/2
  Sum2_NODE18/1 -> Product1_NODE18/1
  Product1_NODE18/1 -> Sum3_NODE18/1
  Int1_NODE18/1 -> Product1_NODE18/2, EMF_NODE18/1(u), WorkSpaceState_NODE18/1
  Sum3_NODE18/1 -> Int1_NODE18/1
  ServiceThr1_NODE18/1 -> EMF_NODE18/2(u0)
  EMF_NODE18/1(y) -> Out1_NODE18/1, WorkSpaceOut_NODE18/1

== system Lombardy/NODE19 ==
  In1 : Inport
  EMF_NODE19 : MATLAB Function  TreatAsAtomicUnit=on
  Gain1_NODE19 : Gain  Gain=-f_NODE19  SaturateOnIntegerOverflow=on  OutDataTypeStr=Inherit: Same as input  ParamDataTypeStr=Inherit: Same as input
  Gain2_NODE19 : Gain  Gain=-r_NODE19  SaturateOnIntegerOverflow=on  OutDataTypeStr=Inherit: Same as input  ParamDataTypeStr=Inherit: Same as input
  Int1_NODE19 : Integrator  InitialCondition=1
  Product1_NODE19 : Product  SaturateOnIntegerOverflow=on  RndMeth=Zero  InputSameDT=on
  ServiceThr1_NODE19 : Constant  Value=th_NODE19
  Set-off1_NODE19 : Constant
  Sum1_NODE19 : Sum  Inputs=|-+  SaturateOnIntegerOverflow=on  InputSameDT=on
  Sum2_NODE19 : Sum  Inputs=|++  SaturateOnIntegerOverflow=on  InputSameDT=on
  Sum3_NODE19 : Sum  Inputs=|+-  SaturateOnIntegerOverflow=on  InputSameDT=on
  WorkSpaceOut_NODE19 : ToWorkspace  VariableName=Out_NODE19
  WorkSpaceState_NODE19 : ToWorkspace  VariableName=State_NODE19
  Out1_NODE19 : Outport
  wires:
  In1/1 -> Gain2_NODE19/1, Sum1_NODE19/1
  Set-off1_NODE19/1 -> Sum1_NODE19/2
  Sum1_NODE19/1 -> Gain1_NODE19/1
  Gain1_NODE19/1 -> Sum2_NODE19/1
  Gain2_NODE19/1 -> Sum2_NODE19/2, Sum3_NODE19/2
  Sum2_NODE19/1 -> Product1_NODE19/1
  Product1_NODE19/1 -> Sum3_NODE19/1
  Int1_NODE19/1 -> Product1_NODE19/2, EMF_NODE19/1(u), WorkSpaceState_NODE19/1
  Sum3_NODE19/1 -> Int1_NODE19/1
  ServiceThr1_NODE19/1 -> EMF_NODE19/2(u0)
  EMF_NODE19/1(y) -> Out1_NODE19/1, WorkSpaceOut_NODE19/1

== system Lombardy/NODE20 ==
  In1 : Inport
  EMF_NODE20 : MATLAB Function  TreatAsAtomicUnit=on
  Gain1_NODE20 : Gain  Gain=-f_NODE20  SaturateOnIntegerOverflow=on  OutDataTypeStr=Inherit: Same as input  ParamDataTypeStr=Inherit: Same as input
  Gain2_NODE20 : Gain  Gain=-r_NODE20  SaturateOnIntegerOverflow=on  OutDataTypeStr=Inherit: Same as input  ParamDataTypeStr=Inherit: Same as input
  Int1_NODE20 : Integrator  InitialCondition=1
  Product1_NODE20 : Product  SaturateOnIntegerOverflow=on  RndMeth=Zero  InputSameDT=on
  ServiceThr1_NODE20 : Constant  Value=th_NODE20
  Set-off1_NODE20 : Constant
  Sum1_NODE20 : Sum  Inputs=|-+  SaturateOnIntegerOverflow=on  InputSameDT=on
  Sum2_NODE20 : Sum  Inputs=|++  SaturateOnIntegerOverflow=on  InputSameDT=on
  Sum3_NODE20 : Sum  Inputs=|+-  SaturateOnIntegerOverflow=on  InputSameDT=on
  WorkSpaceOut_NODE20 : ToWorkspace  VariableName=Out_NODE20
  WorkSpaceState_NODE20 : ToWorkspace  VariableName=State_NODE20
  Out1_NODE20 : Outport
  wires:
  In1/1 -> Gain2_NODE20/1, Sum1_NODE20/1
  Set-off1_NODE20/1 -> Sum1_NODE20/2
  Sum1_NODE20/1 -> Gain1_NODE20/1
  Gain1_NODE20/1 -> Sum2_NODE20/1
  Gain2_NODE20/1 -> Sum2_NODE20/2, Sum3_NODE20/2
  Sum2_NODE20/1 -> Product1_NODE20/1
  Product1_NODE20/1 -> Sum3_NODE20/1
  Int1_NODE20/1 -> Product1_NODE20/2, EMF_NODE20/1(u), WorkSpaceState_NODE20/1
  Sum3_NODE20/1 -> Int1_NODE20/1
  ServiceThr1_NODE20/1 -> EMF_NODE20/2(u0)
  EMF_NODE20/1(y) -> Out1_NODE20/1, WorkSpaceOut_NODE20/1

== system Lombardy/NODE21 ==
  In1 : Inport
  EMF_NODE21 : MATLAB Function  TreatAsAtomicUnit=on
  Gain1_NODE21 : Gain  Gain=-f_NODE21  SaturateOnIntegerOverflow=on  OutDataTypeStr=Inherit: Same as input  ParamDataTypeStr=Inherit: Same as input
  Gain2_NODE21 : Gain  Gain=-r_NODE21  SaturateOnIntegerOverflow=on  OutDataTypeStr=Inherit: Same as input  ParamDataTypeStr=Inherit: Same as input
  Int1_NODE21 : Integrator  InitialCondition=1
  Product1_NODE21 : Product  SaturateOnIntegerOverflow=on  RndMeth=Zero  InputSameDT=on
  ServiceThr1_NODE21 : Constant  Value=th_NODE21
  Set-off1_NODE21 : Constant
  Sum1_NODE21 : Sum  Inputs=|-+  SaturateOnIntegerOverflow=on  InputSameDT=on
  Sum2_NODE21 : Sum  Inputs=|++  SaturateOnIntegerOverflow=on  InputSameDT=on
  Sum3_NODE21 : Sum  Inputs=|+-  SaturateOnIntegerOverflow=on  InputSameDT=on
  WorkSpaceOut_NODE21 : ToWorkspace  VariableName=Out_NODE21
  WorkSpaceState_NODE21 : ToWorkspace  VariableName=State_NODE21
  Out1_NODE21 : Outport
  wires:
  In1/1 -> Gain2_NODE21/1, Sum1_NODE21/1
  Set-off1_NODE21/1 -> Sum1_NODE21/2
  Sum1_NODE21/1 -> Gain1_NODE21/1
  Gain1_NODE21/1 -> Sum2_NODE21/1
  Gain2_NODE21/1 -> Sum2_NODE21/2, Sum3_NODE21/2
  Sum2_NODE21/1 -> Product1_NODE21/1
  Product1_NODE21/1 -> Sum3_NODE21/1
  Int1_NODE21/1 -> Product1_NODE21/2, EMF_NODE21/1(u), WorkSpaceState_NODE21/1
  Sum3_NODE21/1 -> Int1_NODE21/1
  ServiceThr1_NODE21/1 -> EMF_NODE21/2(u0)
  EMF_NODE21/1(y) -> Out1_NODE21/1, WorkSpaceOut_NODE21/1

== system Lombardy/NODE22 ==
  In1 : Inport
  EMF_NODE22 : MATLAB Function  TreatAsAtomicUnit=on
  Gain1_NODE22 : Gain  Gain=-f_NODE22  SaturateOnIntegerOverflow=on  OutDataTypeStr=Inherit: Same as input  ParamDataTypeStr=Inherit: Same as input
  Gain2_NODE22 : Gain  Gain=-r_NODE22  SaturateOnIntegerOverflow=on  OutDataTypeStr=Inherit: Same as input  ParamDataTypeStr=Inherit: Same as input
  Int1_NODE22 : Integrator  InitialCondition=1
  Product1_NODE22 : Product  SaturateOnIntegerOverflow=on  RndMeth=Zero  InputSameDT=on
  ServiceThr1_NODE22 : Constant  Value=th_NODE22
  Set-off1_NODE22 : Constant
  Sum1_NODE22 : Sum  Inputs=|-+  SaturateOnIntegerOverflow=on  InputSameDT=on
  Sum2_NODE22 : Sum  Inputs=|++  SaturateOnIntegerOverflow=on  InputSameDT=on
  Sum3_NODE22 : Sum  Inputs=|+-  SaturateOnIntegerOverflow=on  InputSameDT=on
  WorkSpaceOut_NODE22 : ToWorkspace  VariableName=Out_NODE22
  WorkSpaceState_NODE22 : ToWorkspace  VariableName=State_NODE22
  Out1_NODE22 : Outport
  wires:
  In1/1 -> Gain2_NODE22/1, Sum1_NODE22/1
  Set-off1_NODE22/1 -> Sum1_NODE22/2
  Sum1_NODE22/1 -> Gain1_NODE22/1
  Gain1_NODE22/1 -> Sum2_NODE22/1
  Gain2_NODE22/1 -> Sum2_NODE22/2, Sum3_NODE22/2
  Sum2_NODE22/1 -> Product1_NODE22/1
  Product1_NODE22/1 -> Sum3_NODE22/1
  Int1_NODE22/1 -> Product1_NODE22/2, EMF_NODE22/1(u), WorkSpaceState_NODE22/1
  Sum3_NODE22/1 -> Int1_NODE22/1
  ServiceThr1_NODE22/1 -> EMF_NODE22/2(u0)
  EMF_NODE22/1(y) -> Out1_NODE22/1, WorkSpaceOut_NODE22/1

== system Lombardy/NODE23 ==
  In1 : Inport
  EMF_NODE23 : MATLAB Function  TreatAsAtomicUnit=on
  Gain1_NODE23 : Gain  Gain=-f_NODE23  SaturateOnIntegerOverflow=on  OutDataTypeStr=Inherit: Same as input  ParamDataTypeStr=Inherit: Same as input
  Gain2_NODE23 : Gain  Gain=-r_NODE23  SaturateOnIntegerOverflow=on  OutDataTypeStr=Inherit: Same as input  ParamDataTypeStr=Inherit: Same as input
  Int1_NODE23 : Integrator  InitialCondition=1
  Product1_NODE23 : Product  SaturateOnIntegerOverflow=on  RndMeth=Zero  InputSameDT=on
  ServiceThr1_NODE23 : Constant  Value=th_NODE23
  Set-off1_NODE23 : Constant
  Sum1_NODE23 : Sum  Inputs=|-+  SaturateOnIntegerOverflow=on  InputSameDT=on
  Sum2_NODE23 : Sum  Inputs=|++  SaturateOnIntegerOverflow=on  InputSameDT=on
  Sum3_NODE23 : Sum  Inputs=|+-  SaturateOnIntegerOverflow=on  InputSameDT=on
  WorkSpaceOut_NODE23 : ToWorkspace  VariableName=Out_NODE23
  WorkSpaceState_NODE23 : ToWorkspace  VariableName=State_NODE23
  Out1_NODE23 : Outport
  wires:
  In1/1 -> Gain2_NODE23/1, Sum1_NODE23/1
  Set-off1_NODE23/1 -> Sum1_NODE23/2
  Sum1_NODE23/1 -> Gain1_NODE23/1
  Gain1_NODE23/1 -> Sum2_NODE23/1
  Gain2_NODE23/1 -> Sum2_NODE23/2, Sum3_NODE23/2
  Sum2_NODE23/1 -> Product1_NODE23/1
  Product1_NODE23/1 -> Sum3_NODE23/1
  Int1_NODE23/1 -> Product1_NODE23/2, EMF_NODE23/1(u), WorkSpaceState_NODE23/1
  Sum3_NODE23/1 -> Int1_NODE23/1
  ServiceThr1_NODE23/1 -> EMF_NODE23/2(u0)
  EMF_NODE23/1(y) -> Out1_NODE23/1, WorkSpaceOut_NODE23/1

== system Lombardy/NODE24 ==
  In1 : Inport
  EMF_NODE24 : MATLAB Function  TreatAsAtomicUnit=on
  Gain1_NODE24 : Gain  Gain=-f_NODE24  SaturateOnIntegerOverflow=on  OutDataTypeStr=Inherit: Same as input  ParamDataTypeStr=Inherit: Same as input
  Gain2_NODE24 : Gain  Gain=-r_NODE24  SaturateOnIntegerOverflow=on  OutDataTypeStr=Inherit: Same as input  ParamDataTypeStr=Inherit: Same as input
  Int1_NODE24 : Integrator  InitialCondition=1
  Product1_NODE24 : Product  SaturateOnIntegerOverflow=on  RndMeth=Zero  InputSameDT=on
  ServiceThr1_NODE24 : Constant  Value=th_NODE24
  Set-off1_NODE24 : Constant
  Sum1_NODE24 : Sum  Inputs=|-+  SaturateOnIntegerOverflow=on  InputSameDT=on
  Sum2_NODE24 : Sum  Inputs=|++  SaturateOnIntegerOverflow=on  InputSameDT=on
  Sum3_NODE24 : Sum  Inputs=|+-  SaturateOnIntegerOverflow=on  InputSameDT=on
  WorkSpaceOut_NODE24 : ToWorkspace  VariableName=Out_NODE24
  WorkSpaceState_NODE24 : ToWorkspace  VariableName=State_NODE24
  Out1_NODE24 : Outport
  wires:
  In1/1 -> Gain2_NODE24/1, Sum1_NODE24/1
  Set-off1_NODE24/1 -> Sum1_NODE24/2
  Sum1_NODE24/1 -> Gain1_NODE24/1
  Gain1_NODE24/1 -> Sum2_NODE24/1
  Gain2_NODE24/1 -> Sum2_NODE24/2, Sum3_NODE24/2
  Sum2_NODE24/1 -> Product1_NODE24/1
  Product1_NODE24/1 -> Sum3_NODE24/1
  Int1_NODE24/1 -> Product1_NODE24/2, EMF_NODE24/1(u), WorkSpaceState_NODE24/1
  Sum3_NODE24/1 -> Int1_NODE24/1
  ServiceThr1_NODE24/1 -> EMF_NODE24/2(u0)
  EMF_NODE24/1(y) -> Out1_NODE24/1, WorkSpaceOut_NODE24/1

== system Lombardy/NODE25 ==
  In1 : Inport
  EMF_NODE25 : MATLAB Function  TreatAsAtomicUnit=on
  Gain1_NODE25 : Gain  Gain=-f_NODE25  SaturateOnIntegerOverflow=on  OutDataTypeStr=Inherit: Same as input  ParamDataTypeStr=Inherit: Same as input
  Gain2_NODE25 : Gain  Gain=-r_NODE25  SaturateOnIntegerOverflow=on  OutDataTypeStr=Inherit: Same as input  ParamDataTypeStr=Inherit: Same as input
  Int1_NODE25 : Integrator  InitialCondition=1
  Product1_NODE25 : Product  SaturateOnIntegerOverflow=on  RndMeth=Zero  InputSameDT=on
  ServiceThr1_NODE25 : Constant  Value=th_NODE25
  Set-off1_NODE25 : Constant
  Sum1_NODE25 : Sum  Inputs=|-+  SaturateOnIntegerOverflow=on  InputSameDT=on
  Sum2_NODE25 : Sum  Inputs=|++  SaturateOnIntegerOverflow=on  InputSameDT=on
  Sum3_NODE25 : Sum  Inputs=|+-  SaturateOnIntegerOverflow=on  InputSameDT=on
  WorkSpaceOut_NODE25 : ToWorkspace  VariableName=Out_NODE25
  WorkSpaceState_NODE25 : ToWorkspace  VariableName=State_NODE25
  Out1_NODE25 : Outport
  wires:
  In1/1 -> Gain2_NODE25/1, Sum1_NODE25/1
  Set-off1_NODE25/1 -> Sum1_NODE25/2
  Sum1_NODE25/1 -> Gain1_NODE25/1
  Gain1_NODE25/1 -> Sum2_NODE25/1
  Gain2_NODE25/1 -> Sum2_NODE25/2, Sum3_NODE25/2
  Sum2_NODE25/1 -> Product1_NODE25/1
  Product1_NODE25/1 -> Sum3_NODE25/1
  Int1_NODE25/1 -> Product1_NODE25/2, EMF_NODE25/1(u), WorkSpaceState_NODE25/1
  Sum3_NODE25/1 -> Int1_NODE25/1
  ServiceThr1_NODE25/1 -> EMF_NODE25/2(u0)
  EMF_NODE25/1(y) -> Out1_NODE25/1, WorkSpaceOut_NODE25/1

== system Lombardy/NODE26 ==
  In1 : Inport
  EMF_NODE26 : MATLAB Function  TreatAsAtomicUnit=on
  Gain1_NODE26 : Gain  Gain=-f_NODE26  SaturateOnIntegerOverflow=on  OutDataTypeStr=Inherit: Same as input  ParamDataTypeStr=Inherit: Same as input
  Gain2_NODE26 : Gain  Gain=-r_NODE26  SaturateOnIntegerOverflow=on  OutDataTypeStr=Inherit: Same as input  ParamDataTypeStr=Inherit: Same as input
  Int1_NODE26 : Integrator  InitialCondition=1
  Product1_NODE26 : Product  SaturateOnIntegerOverflow=on  RndMeth=Zero  InputSameDT=on
  ServiceThr1_NODE26 : Constant  Value=th_NODE26
  Set-off1_NODE26 : Constant
  Sum1_NODE26 : Sum  Inputs=|-+  SaturateOnIntegerOverflow=on  InputSameDT=on
  Sum2_NODE26 : Sum  Inputs=|++  SaturateOnIntegerOverflow=on  InputSameDT=on
  Sum3_NODE26 : Sum  Inputs=|+-  SaturateOnIntegerOverflow=on  InputSameDT=on
  WorkSpaceOut_NODE26 : ToWorkspace  VariableName=Out_NODE26
  WorkSpaceState_NODE26 : ToWorkspace  VariableName=State_NODE26
  Out1_NODE26 : Outport
  wires:
  In1/1 -> Gain2_NODE26/1, Sum1_NODE26/1
  Set-off1_NODE26/1 -> Sum1_NODE26/2
  Sum1_NODE26/1 -> Gain1_NODE26/1
  Gain1_NODE26/1 -> Sum2_NODE26/1
  Gain2_NODE26/1 -> Sum2_NODE26/2, Sum3_NODE26/2
  Sum2_NODE26/1 -> Product1_NODE26/1
  Product1_NODE26/1 -> Sum3_NODE26/1
  Int1_NODE26/1 -> Product1_NODE26/2, EMF_NODE26/1(u), WorkSpaceState_NODE26/1
  Sum3_NODE26/1 -> Int1_NODE26/1
  ServiceThr1_NODE26/1 -> EMF_NODE26/2(u0)
  EMF_NODE26/1(y) -> Out1_NODE26/1, WorkSpaceOut_NODE26/1

== system Lombardy/NODE27 ==
  In1 : Inport
  EMF_NODE27 : MATLAB Function  TreatAsAtomicUnit=on
  Gain1_NODE27 : Gain  Gain=-f_NODE27  SaturateOnIntegerOverflow=on  OutDataTypeStr=Inherit: Same as input  ParamDataTypeStr=Inherit: Same as input
  Gain2_NODE27 : Gain  Gain=-r_NODE27  SaturateOnIntegerOverflow=on  OutDataTypeStr=Inherit: Same as input  ParamDataTypeStr=Inherit: Same as input
  Int1_NODE27 : Integrator  InitialCondition=1
  Product1_NODE27 : Product  SaturateOnIntegerOverflow=on  RndMeth=Zero  InputSameDT=on
  ServiceThr1_NODE27 : Constant  Value=th_NODE27
  Set-off1_NODE27 : Constant
  Sum1_NODE27 : Sum  Inputs=|-+  SaturateOnIntegerOverflow=on  InputSameDT=on
  Sum2_NODE27 : Sum  Inputs=|++  SaturateOnIntegerOverflow=on  InputSameDT=on
  Sum3_NODE27 : Sum  Inputs=|+-  SaturateOnIntegerOverflow=on  InputSameDT=on
  WorkSpaceOut_NODE27 : ToWorkspace  VariableName=Out_NODE27
  WorkSpaceState_NODE27 : ToWorkspace  VariableName=State_NODE27
  Out1_NODE27 : Outport
  wires:
  In1/1 -> Gain2_NODE27/1, Sum1_NODE27/1
  Set-off1_NODE27/1 -> Sum1_NODE27/2
  Sum1_NODE27/1 -> Gain1_NODE27/1
  Gain1_NODE27/1 -> Sum2_NODE27/1
  Gain2_NODE27/1 -> Sum2_NODE27/2, Sum3_NODE27/2
  Sum2_NODE27/1 -> Product1_NODE27/1
  Product1_NODE27/1 -> Sum3_NODE27/1
  Int1_NODE27/1 -> Product1_NODE27/2, EMF_NODE27/1(u), WorkSpaceState_NODE27/1
  Sum3_NODE27/1 -> Int1_NODE27/1
  ServiceThr1_NODE27/1 -> EMF_NODE27/2(u0)
  EMF_NODE27/1(y) -> Out1_NODE27/1, WorkSpaceOut_NODE27/1

== system Lombardy/NODE28 ==
  In1 : Inport
  EMF_NODE28 : MATLAB Function  TreatAsAtomicUnit=on
  Gain1_NODE28 : Gain  Gain=-f_NODE28  SaturateOnIntegerOverflow=on  OutDataTypeStr=Inherit: Same as input  ParamDataTypeStr=Inherit: Same as input
  Gain2_NODE28 : Gain  Gain=-r_NODE28  SaturateOnIntegerOverflow=on  OutDataTypeStr=Inherit: Same as input  ParamDataTypeStr=Inherit: Same as input
  Int1_NODE28 : Integrator  InitialCondition=1
  Product1_NODE28 : Product  SaturateOnIntegerOverflow=on  RndMeth=Zero  InputSameDT=on
  ServiceThr1_NODE28 : Constant  Value=th_NODE28
  Set-off1_NODE28 : Constant
  Sum1_NODE28 : Sum  Inputs=|-+  SaturateOnIntegerOverflow=on  InputSameDT=on
  Sum2_NODE28 : Sum  Inputs=|++  SaturateOnIntegerOverflow=on  InputSameDT=on
  Sum3_NODE28 : Sum  Inputs=|+-  SaturateOnIntegerOverflow=on  InputSameDT=on
  WorkSpaceOut_NODE28 : ToWorkspace  VariableName=Out_NODE28
  WorkSpaceState_NODE28 : ToWorkspace  VariableName=State_NODE28
  Out1_NODE28 : Outport
  wires:
  In1/1 -> Gain2_NODE28/1, Sum1_NODE28/1
  Set-off1_NODE28/1 -> Sum1_NODE28/2
  Sum1_NODE28/1 -> Gain1_NODE28/1
  Gain1_NODE28/1 -> Sum2_NODE28/1
  Gain2_NODE28/1 -> Sum2_NODE28/2, Sum3_NODE28/2
  Sum2_NODE28/1 -> Product1_NODE28/1
  Product1_NODE28/1 -> Sum3_NODE28/1
  Int1_NODE28/1 -> Product1_NODE28/2, EMF_NODE28/1(u), WorkSpaceState_NODE28/1
  Sum3_NODE28/1 -> Int1_NODE28/1
  ServiceThr1_NODE28/1 -> EMF_NODE28/2(u0)
  EMF_NODE28/1(y) -> Out1_NODE28/1, WorkSpaceOut_NODE28/1
